simulink model "pubsub_multitask"  (R2020a)
settings: Solver=FixedStepDiscrete  StartTime=0.0  StopTime=10.0  RelTol=1e-3  EnableMultiTasking=on
undefined symbols (not defined in the file): nuttx
libraries: uORBlib x1
settings Model: Creator=asanchez  LastModifiedBy=asanchez
settings SolverCC: ConcurrentTasks=on  AutoInsertRateTranBlk=on
settings OptimizationCC: DefaultParameterBehavior=Inlined  EnhancedBackFolding=on  PassReuseOutputArgsAs=Individual arguments  ZeroExternalMemoryAtStartup=off  ZeroInternalMemoryAtStartup=off  MaxStackSize=64  OptimizeBlockOrder=speed  DifferentSizesBufferReuse=on  OptimizationCustomize=off  EfficientTunableParamExpr=on
settings DebuggingCC: ParameterTunabilityLossMsg=error
settings HardwareCC: ProdLongLongMode=on  TargetBitPerLong=64  TargetBitPerPointer=64  TargetBitPerSizeT=64  TargetBitPerPtrDiffT=64  TargetLongLongMode=on  TargetIntDivRoundTo=Zero  TargetEndianess=LittleEndian  TargetWordSize=64  TargetHWDeviceType=MATLAB Host  HardwareBoardFeatureSet=SoCBlockset
settings SFSimCC: SimGenImportedTypeDefs=on  MATLABDynamicMemAlloc=off
settings RTWCC: Description=Nuttx EC Target  SystemTargetFile=nuttx_ec.tlc  GenCodeOnly=on  GenerateMakefile=off  TemplateMakefile=nuttx_ec.tmf  PostCodeGenCommand=nuttx_ec.onAfterCodeGen(Simulink.ConfigSet, buildInfo)  RTWVerbose=off  Toolchain=AUTOSAR Adaptive | CMake  TargetLang=C++
settings CodeAppCC: ForceParamTrailComments=on  IgnoreCustomStorageClasses=off  MaxIdLength=63  OperatorAnnotations=on  SimulinkDataObjDesc=on  SFDataObjDesc=on  InsertBlockDesc=on
settings STFCustomTargetCC: TargetLibSuffix=.a  TargetLangStandard=C++03 (ISO)  MultiwordLength=256  ConcurrentExecutionCompliant=on  CombineOutputUpdateFcns=on  ERTCustomFileBanners=on  SupportContinuousTime=off  SupportNonInlinedSFcns=off  RemoveResetFunc=on  MATLABClassNameForMDSCustomization=Simulink.SoftwareTarget.ERTCustomization  SystemTargetFile=nuttx_ec.tlc
settings ERTTargetCC: TargetLangStandard=C++03 (ISO)  ParMdlRefBuildCompliant=off  CompOptLevelCompliant=off  ModelStepFunctionPrototypeControlCompliant=off  CPPClassGenCompliant=off  UseToolchainInfoCompliant=off  InlinedParameterPlacement=NonHierarchical  ERTCustomFileTemplate=nuttx_ec_file_process.tlc

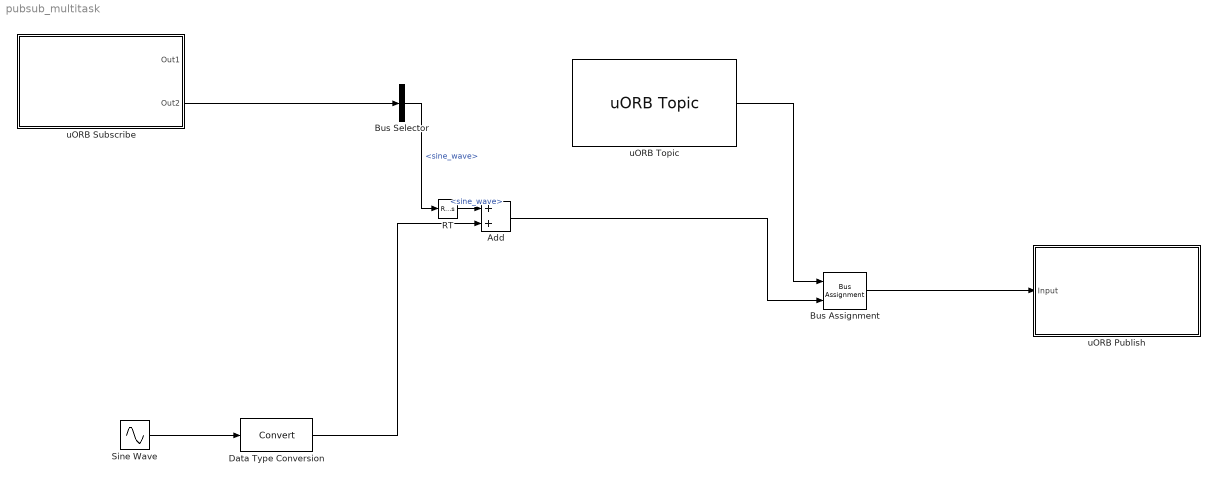
== system pubsub_multitask ==
  Add : Sum
  Bus Assignment : BusAssignment  AssignedSignals=sine_wave
  Bus Selector : BusSelector  OutputSignals=sine_wave
  Data Type Conversion : DataTypeConversion
  RT : RateTransition  OutPortSampleTime=0.01
  Sine Wave : Sin  SampleTime=0.01
  uORB Publish : Subsystem  AncestorBlock=uORBlib/uORB Publish  mask(Nuttx uORB Publish){uORBTopic=aa_tito_prueba, selectInstance=aa_tito_prueba}
      mask prompts: uORBTopic "Topic :"
      mask init:
      | nuttx.internal.block.PublishBlockMask.dispatch('maskInitialize',gcb);
      mask Callback uORBTopic: nuttx.internal.block.PublishBlockMask.dispatch('topicEdit',gcb);
      mask TypeOptions selectInstance: aa_tito_prueba
      mask DialogControl Container4 Prompt: Main
      mask DialogControl topicSelecBtn Prompt: Select
      mask DialogControl topicSelecBtn Callback: nuttx.internal.block.PublishBlockMask.dispatch('topicSelect',gcb);
      mask DialogControl Container5 Prompt: Advanced
      mask Display:
      | color('blue');
      | text(0.2, 0.90, 'Nuttx', 'horizontalAlignment', 'right');
      | color('black');
      | text(0.5, 0.60, 'uORB Publish', 'horizontalAlignment', 'center');
      | if length(uORBTopic) > 20
      |   text(0.95, 0.15, uORBTopic, 'horizontalAlignment', 'right');
      | else
      |   text(0.5, 0.15, uORBTopic, 'horizontalAlignment', 'center');
      | end
      | port_label('input', 1, 'Msg');
  uORB Subscribe : Subsystem  AncestorBlock=uORBlib/uORB Subscribe  mask(Nuttx uORB Read){uORBTopic=aa_tito_prueba, selectInstance=aa_tito_prueba, SampleTime=0.1, BlockingMode=off, BlockTimeout=1e-3}
      mask prompts: uORBTopic "nuttx:blockmask:TopicPrompt"; selectInstance "nuttx:blockmask:SelectInstance"; SampleTime "nuttx:blockmask:SampleTimePrompt"; BlockingMode "Wait until data received"; BlockTimeout "Timeout in seconds:"
      mask init:
      | nuttx.internal.block.SubscribeBlockMask.dispatch('maskInitialize', gcb);
      mask Callback uORBTopic: nuttx.internal.block.SubscribeBlockMask.dispatch('topicEdit', gcb);
      mask TypeOptions selectInstance: aa_tito_prueba
      mask TypeOptions SampleTime: SourceBlock/SampleTime
      mask TypeOptions BlockingMode: SourceBlock/BlockingMode
      mask Callback BlockingMode: nuttx.internal.block.SubscribeBlockMask.dispatch('blockingModeSelect', gcb);
      mask TypeOptions BlockTimeout: SourceBlock/BlockTimeout
      mask DialogControl ContainerMain Prompt: Main
      mask DialogControl topicSelectButton Prompt: Select
      mask DialogControl topicSelectButton Callback: nuttx.internal.block.SubscribeBlockMask.dispatch('topicSelect', gcb);
      mask DialogControl ContainerAdvanced Prompt: Advanced
      mask Display:
      | color('blue');
      | text(0.2, 0.90, 'Nuttx', 'horizontalAlignment', 'right');
      | color('black');
      | text(0.5, 0.60, 'uORB Subscribe', 'horizontalAlignment', 'center');
      | if length(uORBTopic) > 16
      |   text(0.83, 0.15, uORBTopic, 'horizontalAlignment', 'right');
      | else
      |   text(0.5, 0.15, uORBTopic, 'horizontalAlignment', 'center');
      | end
      | port_label('output', 1, 'Status');
      | port_label('output', 2, 'Msg');
  uORB Topic : uORBlib/uORB Topic  uORBTopic=aa_tito_prueba  SampleTime=inf  selectInstance=aa_tito_prueba
      settings: SourceProductName=Nuttx Toolbox Support Package
  wires:
  uORB Topic/1 -> Bus Assignment/1
  Sine Wave/1 -> Data Type Conversion/1
  Data Type Conversion/1 -> Add/2
  Bus Assignment/1 -> uORB Publish/1(Input)
  uORB Subscribe/2(Out2) -> Bus Selector/1
  Bus Selector/1 -> RT/1  "<sine_wave>"
  Add/1 -> Bus Assignment/2
  RT/1 -> Add/1  "<sine_wave>"

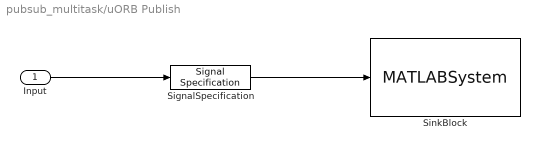
== system pubsub_multitask/uORB Publish ==
  Input : Inport
  SignalSpecification : SignalSpecification  OutDataTypeStr=Bus: nuttx_Bus_aa_tito_prueba  BusOutputAsStruct=on
      settings: LockScale=on
  SinkBlock : MATLABSystem  System=nuttx.internal.block.Publisher  uORBTopic=aa_tito_prueba  MessageQueueLen=1  uORBTopicInstance=aa_tito_prueba  SLBusName=nuttx_Bus_aa_tito_prueba
      mask Type: nuttx.internal.block.Publisher
      mask Display:
      | disp('Publisher');
      | port_label('input',1,'busstruct');
  wires:
  SignalSpecification/1 -> SinkBlock/1
  Input/1 -> SignalSpecification/1

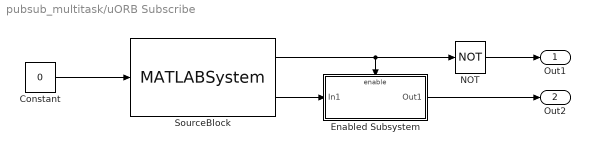
== system pubsub_multitask/uORB Subscribe ==
  Constant : Constant  Value=0  OutDataTypeStr=Bus: nuttx_Bus_aa_tito_prueba
  Enabled Subsystem : Subsystem  TreatAsAtomicUnit=on
  NOT : Logic  Operator=NOT  IconShape=distinctive  AllPortsSameDT=off  OutDataTypeStr=boolean
  SourceBlock : MATLABSystem  InitFcn=nuttx.internal.block.SubscribeBlockMask.dispatch('sysobjInitFcn', gcb);  System=nuttx.internal.block.Subscriber  uORBTopic=aa_tito_prueba  uORBTopicInstance=aa_tito_prueba  SLBusName=nuttx_Bus_aa_tito_prueba  SampleTime=SampleTime  BlockingMode=off  BlockTimeout=BlockTimeout
      mask Type: nuttx.internal.block.Subscriber
      mask Display:
      | disp('Subscriber');
      | port_label('input',1,'busstruct');
      | port_label('output',1,'isNewData');
      | port_label('output',2,'msg');
  Out1 : Outport  SampleTime=0.001
  Out2 : Outport  Port=2
  wires:
  Enabled Subsystem/1(Out1) -> Out2/1
  NOT/1 -> Out1/1
  SourceBlock/1 -> Enabled Subsystem/Enable, NOT/1
  SourceBlock/2 -> Enabled Subsystem/1(In1)
  Constant/1 -> SourceBlock/1

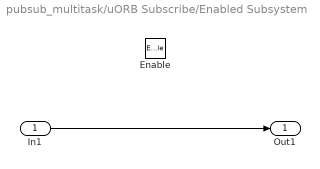
== system pubsub_multitask/uORB Subscribe/Enabled Subsystem ==
  In1 : Inport
  Enable : EnablePort
  Out1 : Outport
  wires:
  In1/1 -> Out1/1
